simulink model "DCC_DTC_v3_5"  (R2023b)
settings: Solver=FixedStepDiscrete  StartTime=0.0  StopTime=0.4  MaxStep=1e-  RelTol=1e-6
undefined symbols (not defined in the file): DiscIntNeverNeededParam
libraries: spsPermanentMagnetSynchronousMachineLib x2, simulink x2, spsDCVoltageSourceLib x1, spsGroundLib x1, spsThreePhaseVIMeasurementLib x1, spsUniversalBridgeLib x1, sps_lib x1
settings Model: Creator=rainy  LastModifiedBy=rainy
settings DataIOCC: ReturnWorkspaceOutputs=off

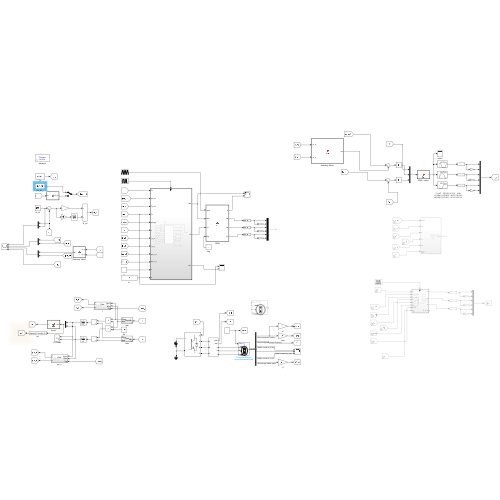
[thumbnail: Simulink's stored preview of the top-level diagram]
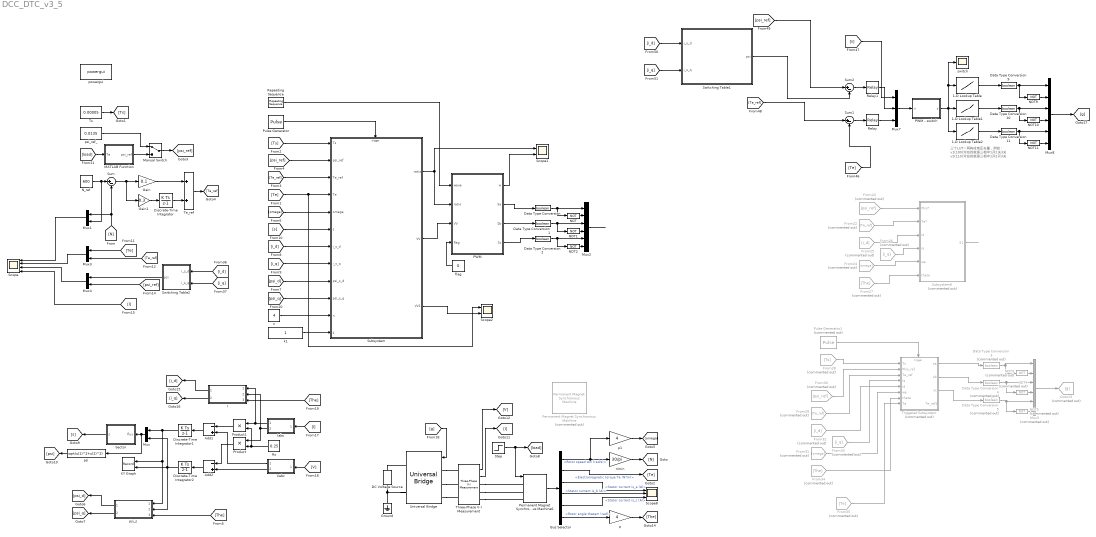
== system DCC_DTC_v3_5 ==
  note: 三个LUT一同构成电压矢量，例如：
      | v1(100)对应的就是三相中1开2关3关
      | v2(110)对应的就是三相中1开2开3关
  1-D Lookup Table : Lookup_n-D  NumberOfTableDimensions=1  BreakpointsForDimension1=[1 2 3 4 5 6]  Table=[1 1 0 0 0 1]  InternalRulePriority=Speed  RndMeth=Simplest
  1-D Lookup Table1 : Lookup_n-D  NumberOfTableDimensions=1  BreakpointsForDimension1=[1 2 3 4 5 6]  Table=[0 1 1 1 0 0]  InternalRulePriority=Speed  RndMeth=Simplest
  1-D Lookup Table2 : Lookup_n-D  NumberOfTableDimensions=1  BreakpointsForDimension1=[1 2 3 4 5 6]  Table=[0 0 0 1 1 1]  InternalRulePriority=Speed  RndMeth=Simplest
  Add1 : Sum  Inputs=-+
  Add2 : Sum  Inputs=-+
  Bus Selector : BusSelector  OutputSignals=Rotor speed wm (rad/s),Electromagnetic torque Te (N*m),Stator current is_a (A),Stator current is_b (A),Stator current is_c (A),Rotor angle thetam (rad)
  DC Voltage Source : spsDCVoltageSourceLib/DC Voltage Source  Amplitude=24  Measurements=Voltage
  Data Type Conversion{,1..2,9..11} (6 alike) : DataTypeConversion  OutDataTypeStr=boolean  SaturateOnIntegerOverflow=off  RndMeth=Floor
  Data Type Conversion3 : DataTypeConversion  Commented=on  OutDataTypeStr=boolean  SaturateOnIntegerOverflow=off  RndMeth=Floor
  Data Type Conversion4 : DataTypeConversion  Commented=on  OutDataTypeStr=boolean  SaturateOnIntegerOverflow=off  RndMeth=Floor
  Data Type Conversion5 : DataTypeConversion  Commented=on  OutDataTypeStr=boolean  SaturateOnIntegerOverflow=off  RndMeth=Floor
  Discrete-Time Integrator : DiscreteIntegrator  SampleTime=-1  ICPrevOutput=DiscIntNeverNeededParam  ICPrevScaledInput=DiscIntNeverNeededParam
  Discrete-Time Integrator1 : DiscreteIntegrator  SampleTime=-1  ICPrevOutput=DiscIntNeverNeededParam  ICPrevScaledInput=DiscIntNeverNeededParam
  Discrete-Time Integrator2 : DiscreteIntegrator  SampleTime=-1  ICPrevOutput=DiscIntNeverNeededParam  ICPrevScaledInput=DiscIntNeverNeededParam
  From22 : From  Commented=on  GotoTag=Te_ref
  From23 : From  Commented=on  GotoTag=psi_ref
  From24 : From  Commented=on  GotoTag=omega
  From25 : From  Commented=on  GotoTag=i_d
  From26 : From  Commented=on  GotoTag=i_q
  From27 : From  Commented=on  GotoTag=The
  From28 : From  Commented=on  GotoTag=Ts
  From29 : From  Commented=on  GotoTag=Te_ref
  From30 : From  Commented=on  GotoTag=psi_ref
  From31 : From  Commented=on  GotoTag=omega
  From32 : From  Commented=on  GotoTag=i_d
  From33 : From  Commented=on  GotoTag=i_q
  From34 : From  Commented=on  GotoTag=The
  From35 : From  Commented=on  GotoTag=Te
  Gain : Gain  Gain=0.1
  Gain1 : Gain  Gain=0.3
  Goto13 : Goto  Commented=on  GotoTag=g
  Ground : spsGroundLib/Ground  LConnTagsString=a
  I : Subsystem  ReferencedSubsystem=Park
  Iabc : Subsystem  ReferencedSubsystem=Clark
  MATLAB Function : MATLAB Function  TreatAsAtomicUnit=on
  Manual Switch : ManualSwitch
  Mux{,1,3..4} (4 alike) : Mux  Inputs=2
  Mux2 : Mux  Inputs=6
  Mux5 : Mux  Commented=on  Inputs=6
  Mux7 : Mux  Inputs=3
  Mux8 : Mux  Inputs=6
  NOT{,1..2,9..11} (6 alike) : Logic  Operator=NOT  IconShape=distinctive  AllPortsSameDT=off  OutDataTypeStr=boolean
  NOT3 : Logic  Commented=on  Operator=NOT  IconShape=distinctive  AllPortsSameDT=off  OutDataTypeStr=boolean
  NOT4 : Logic  Commented=on  Operator=NOT  IconShape=distinctive  AllPortsSameDT=off  OutDataTypeStr=boolean
  NOT5 : Logic  Commented=on  Operator=NOT  IconShape=distinctive  AllPortsSameDT=off  OutDataTypeStr=boolean
  N_ref : Constant  Value=600
  PWM : MATLAB Function  TreatAsAtomicUnit=on
  PWM - switch : MATLAB Function  TreatAsAtomicUnit=on
  Permanent Magnet Synchronous Machine : spsPermanentMagnetSynchronousMachineLib/Permanent Magnet Synchronous Machine  Commented=on  NbPhases=3  FluxDistribution=Sinusoidal  RotorType=Salient-pole  MechanicalLoad=Torque Tm  PresetModel="02:  1.7 Nm 300 Vdc 3750 RPM - 1.7 Nm"  ShowDetailedParameters=on  MeasurementBus=off  Resistance=4.765  Inductance=8.5e-3  dqInductances=[0.0133 0.0147]  La=0.0005  MachineConstant=Flux linkage established by magnets (V.s)  Flux=0.1848  VoltageCst=67.038  TorqueCst=0.5544  Flat=120  Mechanical=[0.0001051 4.047e-05 2 0]  PolePairs=2  InitialConditions=[0 0 0 0]  InitialConditions5ph=[0 0 0 0 0 0]  RefAngle=Aligned with phase A axis (original Park)  IterativeDiscreteModel=Trapezoidal non iterative  TsBlock=-1  TsPowergui=0
  Permanent Magnet Synchronous Machine6 : spsPermanentMagnetSynchronousMachineLib/Permanent Magnet Synchronous Machine  NbPhases=3  FluxDistribution=Sinusoidal  RotorType=Round  MechanicalLoad=Torque Tm  PresetModel=No  ShowDetailedParameters=on  MeasurementBus=off  Resistance=0.25  Inductance=8.5e-3  dqInductances=[8.5e-3,8.5e-3]  La=0.0005  MachineConstant=Flux linkage established by magnets (V.s)  Flux=0.01325  VoltageCst=9.6131  TorqueCst=0.0795  Flat=120  Mechanical=[0.00003 0 4 0]  PolePairs=4  InitialConditions=[0,0, 0,0]  InitialConditions5ph=[0 0 0 0 0 0]  RefAngle=Aligned with phase A axis (original Park)  IterativeDiscreteModel=Trapezoidal non iterative  TsBlock=-1  TsPowergui=0
  Product : Product
  Product1 : Product
  Pulse Generator : DiscretePulseGenerator  PulseType=Time based  Period=0.00005
  Pulse Generator1 : DiscretePulseGenerator  Commented=on  PulseType=Time based  Period=0.00005
  Relay : Relay  OnSwitchValue=0.01  OffSwitchValue=-0.01
  Relay1 : Relay  OnSwitchValue=0.0002  OffSwitchValue=-0.0002
  Repeating Sequence : simulink/Sources/Repeating Sequence  rep_seq_t=[0 0.000025 0.00005]  rep_seq_y=[0 1 0]
  Rs : Constant  Value=0.25
  Scope : Scope  NumInputPorts=4
  Scope1 : Scope  NumInputPorts=2
  Scope2 : Scope  NumInputPorts=2
  Scope8 : Scope  NumInputPorts=3
  Sector : MATLAB Function  TreatAsAtomicUnit=on
  Step : Step  Time=0.2  After=0.5  SampleTime=0
  Subsystem : Subsystem
  Subsystem6 : Subsystem  Commented=on
  Sum : Sum  Inputs=|+-
  Sum1 : Sum  Inputs=|+-
  Sum2 : Sum  Inputs=|+-
  Switching Table1 : MATLAB Function  TreatAsAtomicUnit=on
  Switching Table2 : MATLAB Function  TreatAsAtomicUnit=on
  Te_ref : Sum
  Three-Phase V-I Measurement : spsThreePhaseVIMeasurementLib/Three-Phase V-I Measurement  VoltageMeasurement=phase-to-ground  SetLabelV=off  LabelV=Vabc  Vpu=off  VpuLL=off  CurrentMeasurement=yes  SetLabelI=off  LabelI=Iabc  Ipu=off  Pbase=100e6  Vbase=500e3  OutputType=Complex  PhasorSimulation=off  PSBequivalent=0
  Triggered Subsystem : Subsystem  Commented=on  TreatAsAtomicUnit=on
  Ts : Constant  Value=0.00005
  Universal Bridge : spsUniversalBridgeLib/Universal Bridge  Arms=3  SnubberResistance=1e5  SnubberCapacitance=inf  Device=IGBT / Diodes  Ron=1e-3  Lon=0  ForwardVoltages="[  0  0  ]"  ForwardVoltage=0  GTOparameters=[ 10e-6 , 20e-6 ]  IGBTparameters=[ 1e-6 , 2e-6 ]  Measurements=None  Measurements_2=None  converterType=Rectifier
  Vabc : Subsystem  ReferencedSubsystem=Clark
  XY Graph : Record  FileSettingsInternal="{\"entries\":[{\"content\":{\"excelSettings\":{\"content\":{},\"type\":\"Streamout.ExcelSettings\"}},\"type\":\"Streamout.FileSettingStorage\",\"uuid\":\"\"}],\"packageUris\":[\"http:\\/\\/schema.mathworks.com\\/mf0\\/streamout_blocks\\/R2020a\"],\"version\":\"1.0\"}"  Layout=[1 1]  SignalsInternal="{\"entries\":[{\"content\":{\"signals\":[{\"content\":{\"blockPath\":[],\"dimensions\":[1],\"domain\":\"\",\"lineColor\":\"#a2142f\",\"plots\":[1],\"port\":1,\"sid\":[\"\"],\"signalID\":13639,\"signalName\":\"Discrete-Time\\nIntegrator1\"},\"type\":\"RecordBlkView.Signal\",\"uuid\":\"\"},{\"content\":{\"blockPath\":[],\"dimensions\":[1],\"domain\":\"\",\"lineColor\":\"#139fff\",\"plots\":[1],\"port\":2,\"sid\":[\"\"],\"signalID\":13643,\"signalName\":\"Discrete-Time\\nIntegrator2\"},\"type\":\"RecordBlkView.Signal\",\"uuid\":\"\"}]},\"type\":\"RecordBlkView.InputSignals\",\"uuid\":\"\"}],\"packageUris\":[\"http:\\/\\/schema.mathworks.com\\/mf0\\/streamout_blocks\\/R2020a\"],\"version\":\"1.0\"}"  VisualizationBindings="{\"xyplotplugin\":{\"info\":[{\"series\":[{\"bindingParametersList\":[{\"parameter\":\"X-Axis\",\"signalID\":13639,\"signalName\":\"Discrete-Time\\nIntegrator1\"},{\"parameter\":\"Y-Axis\",\"signalID\":13643,\"signalName\":\"Discrete-Time\\nIntegrator2\"}],\"seriesID\":35459}],\"subplotID\":1}]}}"  CompatibilityTag=XY  st=-1
  flag : Constant  Value=0
  k1 : Constant
  n : Constant  Value=4
  p : Gain  Gain=4
  p1 : Gain  Gain=4
  powergui : sps_lib/powergui  Priority=1  SimulationMode=Discrete  SampleTime=1e-6  frequency=60  Iterations=50  frequencyindice=0  Pbase=100e6  ErrMax=1e-4  UnitsV=kV  UnitsW=MW  buscounter=0  FunctionMessages=off  echomessages=off  EnableUseOfTLC=off  CurrentSourceSwitches=off  DisableSnubberDevices=off  DisableRonSwitches=off  DisableVfSwitches=off  DisplayEquations=off  AutomaticDiscreteSolvers=off  SolverType=Tustin/Backward Euler (TBE)  Interpol=off  ExternalGateDelay=off  methode=off  Ts=100  x0status=blocks  SPID=on  SwTol=0  HookPort=off  NonlinearTolerance=1e-4  nMaxIteration=100  ContinueOnMaxIteration=off  RestoreLinks=warning  ResistiveCurrentMeasurement=off  Frange=[0:2:500]  Ylog=off  Xlog=on  ShowGrid=off  save=off  variable=ZData  structure=0  ZoomFFT=off  StartTime=0.0  cycles=1  DisplayStyle=1  fundamental=60  FreqAxis=off  MaxFrequency=1000  frequencyindicesteady=1  RmsSteady=1  display=off
  psi : Fcn  Expr=sqrt(u(1)^2+u(2)^2)
  psi_ref_ : Constant  Value=0.0135
  psi_s : Subsystem  ReferencedSubsystem=Park
  r/min : Gain  Gain=30/pi
  switch : Scope
  wires:
  N_ref/1 -> Mux1/2, Sum/1
  Sum/1 -> Gain/1, Gain1/1
  Gain1/1 -> Discrete-Time Integrator/1
  Gain/1 -> Te_ref/1
  Bus Selector/1 -> p1/1, r/min/1  "<Rotor speed wm (rad/s)>"
  r/min/1 -> [N]
  [N] -> Sum/2, Mux1/1
  NOT1/1 -> Mux2/4
  Data Type Conversion2/1 -> NOT2/1, Mux2/5
  NOT2/1 -> Mux2/6
  Data Type Conversion/1 -> NOT/1, Mux2/1
  NOT/1 -> Mux2/2
  Data Type Conversion1/1 -> NOT1/1, Mux2/3
  Iabc/1 -> I/1, Product1/1
  Iabc/2 -> Product/1, I/2
  Rs/1 -> Product/2, Product1/2
  Product1/1 -> Add1/1
  Vabc/1 -> Add1/2
  Product/1 -> Add2/1
  Vabc/2 -> Add2/2
  Add2/1 -> Discrete-Time Integrator2/1
  Add1/1 -> Discrete-Time Integrator1/1
  Ts/1 -> [Ts]
  Mux/1 -> psi/1, Sector/1(flux)
  Bus Selector/2 -> [Te]  "<Electromagnetic torque Te (N*m)>"
  [Te] -> Scope2/1, Subsystem/4(Te)
  Three-Phase V-I Measurement/2 -> [I]
  Discrete-Time Integrator/1 -> Te_ref/2
  PWM/4(Sc) -> Data Type Conversion2/1
  PWM/3(Sb) -> Data Type Conversion1/1
  PWM/2(Sa) -> Data Type Conversion/1
  [Ts] -> Subsystem/1(Ts)
  [psi_ref] -> Subsystem/2(psi_ref)
  Repeating Sequence/1 -> PWM/1(wave)
  Pulse Generator/1 -> Subsystem/Trigger
  n/1 -> Subsystem/11(n)
  flag/1 -> PWM/4(flag)
  Bus Selector/3 -> Scope8/1  "<Stator current is_a (A)>"
  Bus Selector/4 -> Scope8/2  "<Stator current is_b (A)>"
  Bus Selector/5 -> Scope8/3  "<Stator current is_c (A)>"
  Step/1 -> Permanent Magnet Synchronous Machine6/1, [load]
  Subsystem/1(ratio) -> PWM/2(ratio), Scope1/1
  Subsystem/2(VV) -> PWM/3(VV)
  Te_ref/1 -> [Te_ref]
  [Te_ref] -> Subsystem/3(Te_ref)
  [omega] -> Subsystem/5(omega)
  [i_d] -> Subsystem/7(i_s_d)
  [i_q] -> Subsystem/8(i_s_q)
  Sector/1(s) -> [s]
  [s] -> Subsystem/6(s)
  PWM/1(w) -> Scope1/2
  psi/1 -> [psi]
  Mux1/1 -> Scope/1
  Mux3/1 -> Scope/2
  Mux4/1 -> Scope/3
  [I] -> Scope/4
  [Te] -> Mux3/1
  Switching Table2/1(psi) -> Mux4/1
  [Te_ref] -> Mux3/2
  [psi_ref] -> Mux4/2
  Three-Phase V-I Measurement/1 -> [V]
  [I] -> Iabc/1
  [V] -> Vabc/1
  Mux2/1 -> ?
  [g] -> Universal Bridge/1
  Bus Selector/6 -> p/1  "<Rotor angle thetam (rad)>"
  p/1 -> [The]
  [The] -> I/3
  I/2 -> [i_q]
  I/1 -> [i_d]
  p1/1 -> [omega]
  k1/1 -> Subsystem/12(k)
  psi_s/1 -> [psi_d]
  Discrete-Time Integrator1/1 -> XY Graph/1, psi_s/1, Mux/1
  psi_s/2 -> [psi_q]
  [The] -> psi_s/3
  Discrete-Time Integrator2/1 -> psi_s/2, XY Graph/2, Mux/2
  [psi_q] -> Subsystem/10(psi_s_q)
  [psi_d] -> Subsystem/9(psi_s_d)
  [load] -> MATLAB Function/1(Te)
  psi_ref_/1 -> Manual Switch/1
  MATLAB Function/1(psi_ref) -> Manual Switch/2
  Manual Switch/1 -> [psi_ref]
  From23/1 -> Subsystem6/1(Phis*)
  From22/1 -> Subsystem6/2(Te*)
  From25/1 -> Subsystem6/3(id)
  From24/1 -> Subsystem6/5(we)
  From26/1 -> Subsystem6/4(iq)
  From27/1 -> Subsystem6/6("theta ")
  NOT5/1 -> Mux5/6
  Triggered Subsystem/2(sb) -> Data Type Conversion4/1
  Data Type Conversion5/1 -> NOT5/1, Mux5/5
  Data Type Conversion4/1 -> NOT4/1, Mux5/3
  Triggered Subsystem/3(sc) -> Data Type Conversion5/1
  Triggered Subsystem/1(sa) -> Data Type Conversion3/1
  NOT4/1 -> Mux5/4
  Data Type Conversion3/1 -> NOT3/1, Mux5/1
  NOT3/1 -> Mux5/2
  Pulse Generator1/1 -> Triggered Subsystem/Trigger
  From28/1 -> Triggered Subsystem/1(Ts)
  From31/1 -> Triggered Subsystem/6(we)
  From29/1 -> Triggered Subsystem/3(Te_ref)
  From34/1 -> Triggered Subsystem/7(theta)
  From32/1 -> Triggered Subsystem/5(id)
  From30/1 -> Triggered Subsystem/2(Phis_ref)
  From33/1 -> Triggered Subsystem/4(iq)
  Permanent Magnet Synchronous Machine6/1 -> Bus Selector/1
  Subsystem6/1(S1) -> ?
  Mux5/1 -> Goto13/1
  Subsystem/3(VV1) -> Scope2/2
  From35/1 -> Triggered Subsystem/8(Te)
  PWM - switch/1(y) -> 1-D Lookup Table2/1, switch/1, 1-D Lookup Table/1, 1-D Lookup Table1/1
  Relay1/1 -> Mux7/2
  Relay/1 -> Mux7/3
  Data Type Conversion9/1 -> NOT9/1, Mux8/1
  1-D Lookup Table2/1 -> Data Type Conversion11/1
  Mux7/1 -> PWM - switch/1(u)
  Sum2/1 -> Relay1/1
  1-D Lookup Table/1 -> Data Type Conversion9/1
  NOT10/1 -> Mux8/4
  NOT9/1 -> Mux8/2
  Data Type Conversion10/1 -> Mux8/3, NOT10/1
  1-D Lookup Table1/1 -> Data Type Conversion10/1
  Sum1/1 -> Relay/1
  Data Type Conversion11/1 -> Mux8/5, NOT11/1
  NOT11/1 -> Mux8/6
  Mux8/1 -> [g]
  [s] -> Mux7/1
  [psi_ref] -> Sum2/1
  [Te] -> Sum1/2
  [Te_ref] -> Sum1/1
  Switching Table1/1(psi) -> Sum2/2
  [i_d] -> Switching Table1/1(i_s_d)
  [i_q] -> Switching Table1/2(i_s_q)
  [i_d] -> Switching Table2/1(i_s_d)
  [i_q] -> Switching Table2/2(i_s_q)
  connections:
  Universal Bridge/RConn2 -- DC Voltage Source/LConn1 -- Ground/LConn1
  Universal Bridge/LConn3 -- Three-Phase V-I Measurement/LConn3
  Universal Bridge/LConn1 -- Three-Phase V-I Measurement/LConn1
  Universal Bridge/LConn2 -- Three-Phase V-I Measurement/LConn2
  DC Voltage Source/RConn1 -- Universal Bridge/RConn1
  Three-Phase V-I Measurement/RConn1 -- Permanent Magnet Synchronous Machine6/LConn1
  Three-Phase V-I Measurement/RConn2 -- Permanent Magnet Synchronous Machine6/LConn2
  Three-Phase V-I Measurement/RConn3 -- Permanent Magnet Synchronous Machine6/LConn3

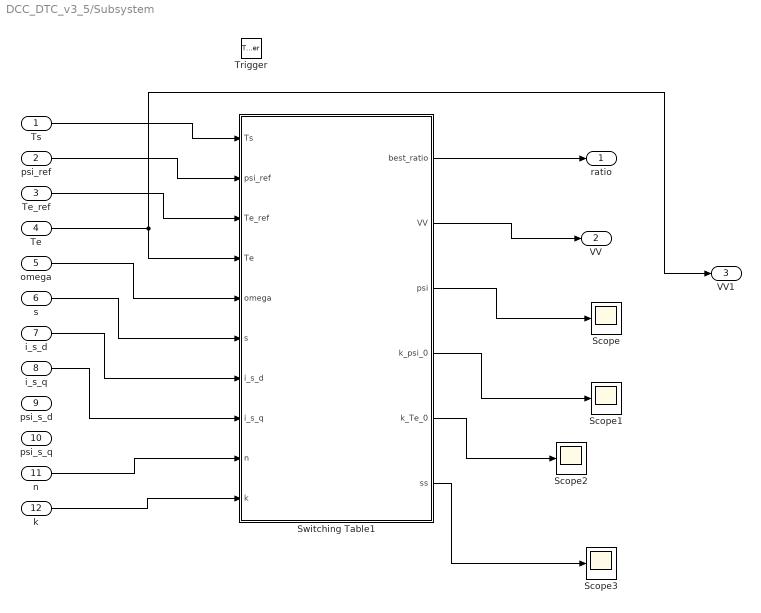
== system DCC_DTC_v3_5/Subsystem ==
  Ts : Inport
  psi_ref : Inport  Port=2
  Te_ref : Inport  Port=3
  Te : Inport  Port=4
  omega : Inport  Port=5
  s : Inport  Port=6
  i_s_d : Inport  Port=7
  i_s_q : Inport  Port=8
  psi_s_d : Inport  Port=9
  psi_s_q : Inport  Port=10
  n : Inport  Port=11
  k : Inport  Port=12
  Trigger : TriggerPort  VariantControl=(inherit)  PortDimensions=1
  Scope{,1..3} (4 alike) : Scope
  Switching Table1 : MATLAB Function  TreatAsAtomicUnit=on
  ratio : Outport
  VV : Outport  Port=2
  VV1 : Outport  Port=3
  wires:
  Ts/1 -> Switching Table1/1(Ts)
  psi_ref/1 -> Switching Table1/2(psi_ref)
  Te_ref/1 -> Switching Table1/3(Te_ref)
  Te/1 -> Switching Table1/4(Te), VV1/1
  omega/1 -> Switching Table1/5(omega)
  s/1 -> Switching Table1/6(s)
  i_s_q/1 -> Switching Table1/8(i_s_q)
  Switching Table1/1(best_ratio) -> ratio/1
  k/1 -> Switching Table1/10(k)
  n/1 -> Switching Table1/9(n)
  Switching Table1/2(VV) -> VV/1
  i_s_d/1 -> Switching Table1/7(i_s_d)
  Switching Table1/3(psi) -> Scope/1
  Switching Table1/4(k_psi_0) -> Scope1/1
  Switching Table1/5(k_Te_0) -> Scope2/1
  Switching Table1/6(ss) -> Scope3/1

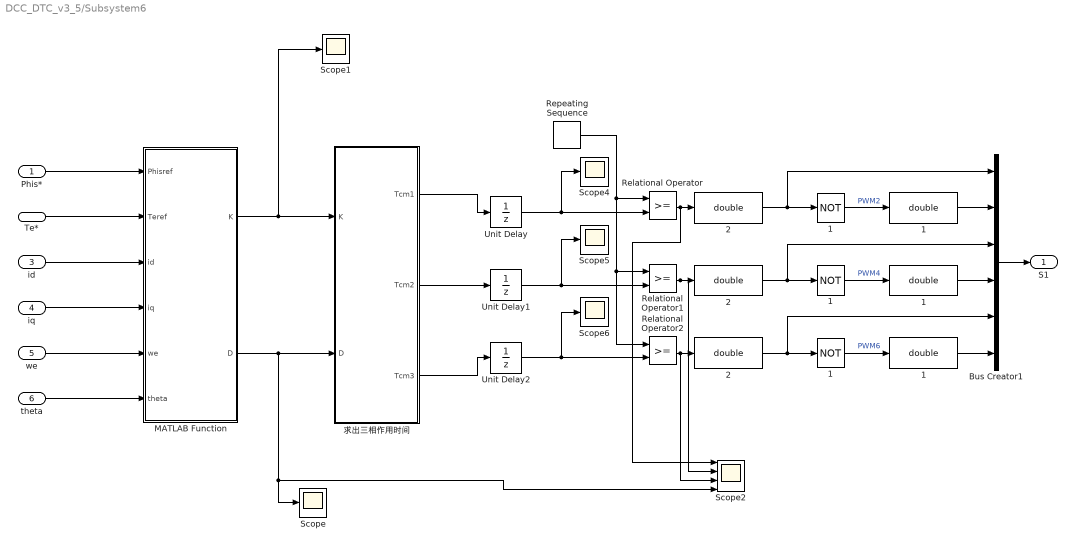
== system DCC_DTC_v3_5/Subsystem6 ==
  Phis* : Inport
  Te* : Inport  Port=2
  id : Inport  Port=3
  iq : Inport  Port=4
  we : Inport  Port=5
  "theta " : Inport  Port=6
  "         1" : DataTypeConversion  OutDataTypeStr=double  SaturateOnIntegerOverflow=off  RndMeth=Floor
  "         2" : DataTypeConversion  OutDataTypeStr=double  SaturateOnIntegerOverflow=off  RndMeth=Floor
  "       1" : Logic  Operator=NOT  AllPortsSameDT=off  OutDataTypeStr=boolean
  "     1" : DataTypeConversion  OutDataTypeStr=double  SaturateOnIntegerOverflow=off  RndMeth=Floor
  "     2" : DataTypeConversion  OutDataTypeStr=double  SaturateOnIntegerOverflow=off  RndMeth=Floor
  "   1" : Logic  Operator=NOT  AllPortsSameDT=off  OutDataTypeStr=boolean
  "  1" : DataTypeConversion  OutDataTypeStr=double  SaturateOnIntegerOverflow=off  RndMeth=Floor
  "  2" : DataTypeConversion  OutDataTypeStr=double  SaturateOnIntegerOverflow=off  RndMeth=Floor
  " 1" : Logic  Operator=NOT  AllPortsSameDT=off  OutDataTypeStr=boolean
  Bus Creator1 : BusCreator  Inputs=6
  MATLAB Function : MATLAB Function  TreatAsAtomicUnit=on
  Relational Operator : RelationalOperator  OutDataTypeStr=boolean  RndMeth=Simplest  InputSameDT=off
  Relational Operator1 : RelationalOperator  OutDataTypeStr=boolean  RndMeth=Simplest  InputSameDT=off
  Relational Operator2 : RelationalOperator  OutDataTypeStr=boolean  RndMeth=Simplest  InputSameDT=off
  Repeating Sequence : simulink/Sources/Repeating Sequence  rep_seq_t=[0 0.000025 0.00005]  rep_seq_y=[0 0.000025 0]
  Scope{,1,4..6} (5 alike) : Scope
  Scope2 : Scope  NumInputPorts=4
  Unit Delay : UnitDelay  SampleTime=0.00005  HasFrameUpgradeWarning=on
  Unit Delay1 : UnitDelay  SampleTime=0.00005  HasFrameUpgradeWarning=on
  Unit Delay2 : UnitDelay  SampleTime=0.00005  HasFrameUpgradeWarning=on
  求出三相作用时间 : MATLAB Function  TreatAsAtomicUnit=on
  S1 : Outport  VectorParamsAs1DForOutWhenUnconnected=off
  wires:
  Phis*/1 -> MATLAB Function/1(Phisref)
  Te*/1 -> MATLAB Function/2(Teref)
  id/1 -> MATLAB Function/3(id)
  iq/1 -> MATLAB Function/4(iq)
  we/1 -> MATLAB Function/5(we)
  "theta "/1 -> MATLAB Function/6(theta)
  MATLAB Function/1(K) -> Scope1/1, 求出三相作用时间/1(K)
  MATLAB Function/2(D) -> Scope2/4, Scope/1, 求出三相作用时间/2(D)
  求出三相作用时间/3(Tcm3) -> Unit Delay2/1
  "   1"/1 -> "     1"/1  "PWM4"
  "     2"/1 -> Bus Creator1/3, "   1"/1
  "     1"/1 -> Bus Creator1/4
  求出三相作用时间/1(Tcm1) -> Unit Delay/1
  " 1"/1 -> "  1"/1  "PWM2"
  Repeating Sequence/1 -> Relational Operator2/1, Relational Operator1/1, Relational Operator/1
  Relational Operator/1 -> Scope2/1, "  2"/1
  Relational Operator1/1 -> Scope2/2, "     2"/1
  求出三相作用时间/2(Tcm2) -> Unit Delay1/1
  "  1"/1 -> Bus Creator1/2
  "         2"/1 -> Bus Creator1/5, "       1"/1
  Relational Operator2/1 -> Scope2/3, "         2"/1
  "       1"/1 -> "         1"/1  "PWM6"
  "  2"/1 -> Bus Creator1/1, " 1"/1
  Bus Creator1/1 -> S1/1
  "         1"/1 -> Bus Creator1/6
  Unit Delay/1 -> Relational Operator/2, Scope4/1
  Unit Delay1/1 -> Scope5/1, Relational Operator1/2
  Unit Delay2/1 -> Relational Operator2/2, Scope6/1

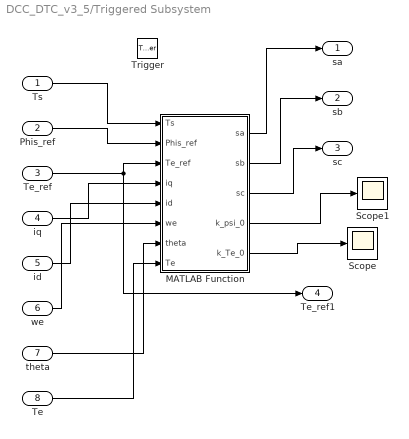
== system DCC_DTC_v3_5/Triggered Subsystem ==
  Ts : Inport
  Phis_ref : Inport  Port=2
  Te_ref : Inport  Port=3
  iq : Inport  Port=4
  id : Inport  Port=5
  we : Inport  Port=6
  theta : Inport  Port=7
  Te : Inport  Port=8
  Trigger : TriggerPort  VariantControl=(inherit)
  MATLAB Function : MATLAB Function  TreatAsAtomicUnit=on
  Scope : Scope
  Scope1 : Scope
  sa : Outport
  sb : Outport  Port=2
  sc : Outport  Port=3
  Te_ref1 : Outport  Port=4
  wires:
  Phis_ref/1 -> MATLAB Function/2(Phis_ref)
  Te_ref/1 -> Te_ref1/1, MATLAB Function/3(Te_ref)
  iq/1 -> MATLAB Function/4(iq)
  id/1 -> MATLAB Function/5(id)
  we/1 -> MATLAB Function/6(we)
  theta/1 -> MATLAB Function/7(theta)
  MATLAB Function/1(sa) -> sa/1
  MATLAB Function/2(sb) -> sb/1
  MATLAB Function/3(sc) -> sc/1
  Ts/1 -> MATLAB Function/1(Ts)
  Te/1 -> MATLAB Function/8(Te)
  MATLAB Function/5(k_Te_0) -> Scope/1
  MATLAB Function/4(k_psi_0) -> Scope1/1

== matlab function DCC_DTC_v3_5/PWM - switch ==
  data: u input; y output
function y = fcn(u)

% u(1) 扇区
% u(2) 磁链
% u(3) 转矩

V_Table=[5 6 1 2 3 4;3 4 5 6 1 2;6 1 2 3 4 5;2 3 4 5 6 1];
x=2*u(2)+u(3)+1;

y = V_Table(x, u(1));

== matlab function DCC_DTC_v3_5/Switching Table2 ==
  data: i_s_d input; i_s_q input; psi output
function psi = fcn(i_s_d, i_s_q)

% 给定的参数值
p = 4;
R_s = 0.25;
L_d = 0.0005;
L_q = 0.0005;
V = 24;
psi_f = 0.01325;

psi_r = psi_f + 1i*0;
psi_s_d = L_d*i_s_d + psi_f;
psi_s_q = L_q*i_s_q;

i_s = i_s_d + 1i*i_s_q;
psi_s = psi_s_d + 1i*psi_s_q;


% 计算零电压矢量下变化率
psi = sqrt(psi_s_d^2 +psi_s_q^2)

== matlab function DCC_DTC_v3_5/Switching Table1 ==
  data: i_s_d input; i_s_q input; psi output
function psi = fcn(i_s_d, i_s_q)

% 给定的参数值
p = 4;
R_s = 0.25;
L_d = 0.0005;
L_q = 0.0005;
V = 24;
psi_f = 0.01325;

psi_r = psi_f + 1i*0;
psi_s_d = L_d*i_s_d + psi_f;
psi_s_q = L_q*i_s_q;

i_s = i_s_d + 1i*i_s_q;
psi_s = psi_s_d + 1i*psi_s_q;


% 计算零电压矢量下变化率
psi = sqrt(psi_s_d^2 +psi_s_q^2)

== matlab function DCC_DTC_v3_5/Sector ==
  data: flux input; s output
function s = fcn(flux)

% 将\psi_{\aplha}和\psi_{\beta}分解为三相
a1 = flux(1);
b1 = flux(1)*(-0.5) + sqrt(3)/2*flux(2);
c1 = flux(1)*(-0.5) - sqrt(3)/2*flux(2);

% a1 > 0，有扇区126
% b1 > 0，有扇区234
% c1 > 0，有扇区456
% n为a1 b1 c1中>0的个数，0 < n < 3
% 
% a b c | s
%-------|---
% 1 1 0 | 2
% 1 0 1 | 6
% 1 0 0 | 1
% 0 1 1 | 4
% 0 1 0 | 3
% 0 0 1 | 5

if(flux(2) == 0)
    N = 4;
else
    if(a1 > 0)
        a = 1;
    else
        a = 0;
    end
    
    if(b1 > 0)
        b = 1;
    else
        b = 0;
    end
    
    if(c1 > 0)
        c = 1;
    else
        c = 0;
    end
    
    N = 4*a+2*b+c;
end

% if(N==0 || N==7)
%     N = 4;
% end

Sector_table=[5 3 4 1 6 2];

s = Sector_table(N);

== matlab function DCC_DTC_v3_5/PWM ==
  data: w output; wave input; ratio input; VV input; Sa output; Sb output; Sc output; flag input
function [w, Sa, Sb, Sc] = fcn(wave, ratio, VV, flag)

sw = [1 0 0; 1 1 0; 0 1 0; 0 1 1; 0 0 1; 1 0 1];

if(VV<1 || VV>6)
    VV = 1;
end

if(wave >= 1 - ratio || flag == 0)
    Sa= sw(VV, 1);
    Sb= sw(VV, 2);
    Sc= sw(VV, 3);
    w = 1;
else
    Sa = 0;
    Sb = 0;
    Sc = 0;
    w = 0;
end

== matlab function DCC_DTC_v3_5/Subsystem6/求出三相作用时间 ==
  settings: updateMethod=DISCRETE  sampleTime=0.00005
  data: K input; Tcm1 output; D input; Tcm2 output; Tcm3 output
function [Tcm1,Tcm2,Tcm3] = fcn(K,D)

Ts=0.00005;

T1=D*Ts/2;
T2=T1;
Ta=(Ts-T1-T2)/4;
Tb=Ta+T1/2;
Tc=Tb+T2/2;
Tcm1=1;
Tcm2=1;
Tcm3=1;

if(K==1)
    Tcm1=Tc;Tcm2=Tc;Tcm3=Tc;
end
if(K==2) 
    Tcm1=Ta;Tcm2=Tc;Tcm3=Tc;
end
if(K==3) 
    Tcm1=Ta;Tcm2=Ta;Tcm3=Tc;
end
if(K==4) 
    Tcm1=Tc;Tcm2=Ta;Tcm3=Tc;
end
if(K==5) 
    Tcm1=Tc;Tcm2=Ta;Tcm3=Ta;
end
if(K==6) 
    Tcm1=Tc;Tcm2=Tc;Tcm3=Ta;
end
if(K==7) 
    Tcm1=Ta;Tcm2=Tc;Tcm3=Ta;
end
if(K==8)
    Tcm1=Ta;Tcm2=Ta;Tcm3=Ta;
end

== matlab function DCC_DTC_v3_5/Subsystem/Switching Table1 ==
  data: best_ratio output; Ts input; psi_ref input; Te_ref input; Te input; VV output; omega input; s input; i_s_d input; i_s_q input; n input; k input; psi output; k_psi_0 output; k_Te_0 output; ss output
function [best_ratio, VV, psi, k_psi_0, k_Te_0, ss]= fcn(Ts, psi_ref, Te_ref, Te, omega, s, i_s_d, i_s_q, n, k)

% 给定的参数值
p = 4;
R_s = 0.25;
L_d = 0.0005;
L_q = 0.0005;
V = 24;
psi_f = 0.01325;

psi_r = psi_f + 1i*0;
psi_s_d = L_d*i_s_d + psi_f;
psi_s_q = L_q*i_s_q;

i_s = i_s_d + 1i*i_s_q;
psi_s = psi_s_d + 1i*psi_s_q;


% 计算零电压矢量下变化率
psi = sqrt(psi_s_d^2 +psi_s_q^2);
k_psi_0 = -R_s/psi*real(psi_s'*i_s); % 零电压矢量时磁链变化率
% k_psi_1 = 1/psi*real(psi_s'*u_s) + k_psi_0; % 非零电压矢量时磁链变化率

k_Te_0 = -3/2*p*(1/L_q-1/L_d)*omega*real(psi_s^2) + ...
    3/4*p*R_s*(1/L_d^2-1/L_q^2)*imag(psi_s^2) - ...
    3/2*p/L_d*(R_s/L_d*imag(psi_s*psi_r) + omega*real(psi_s*psi_r)); % 零电压矢量时转矩变化率
ss = psi_s*psi_r;
% k_Te_1 = 3/2*p*(1/L_q-1/L_d)*imag(u_s*psi_s) + 3/2*p/L_d*imag(u_s*psi_r) + k_Te_0;  % 非零电压矢量时转矩变化率



% 选择电压矢量
Te1 = Te + k_Te_0*Ts;
psi1 = psi + k_psi_0*Ts;

if(Te_ref > Te1)
    if(psi_ref > psi)
        VV = s+1;
    else
        VV = s+2;
    end
else
    if(psi_ref > psi)
        VV = s-1;
    else
        VV = s-2;
    end
end

if(VV < 1)
    VV = VV+6;
end
if(VV > 6)
    VV = VV-6;
end


% MPTC
u_s = cos(pi/6*(VV-1))*V + 1i*sin(pi/6*(VV-1))*V;
k_psi_1 = 1/psi*real(psi_s'*u_s) + k_psi_0; % 非零电压矢量时磁链变化率
k_Te_1 = 3/2*p*(1/L_q-1/L_d)*imag(u_s*psi_s) + 3/2*p/L_d*imag(u_s*psi_r) + k_Te_0;  % 非零电压矢量时转矩变化率

g_min = Inf;
best_ratio = 1;

d_Te = 0;
d_psi = 0;

for i=1:n+1
    ratio = (i-1)*1/n;

    Te1_ = Te + Ts*ratio*k_Te_1 + Ts*(1-ratio)*k_Te_0;
    psi_s1 = psi_s + Ts*ratio*k_psi_1 + Ts*(1-ratio)*k_psi_0;

    d_Te = abs(Te_ref - Te1_);
    d_psi = k*abs(psi_ref - abs(psi_s1));

    g = d_Te + d_psi;

    if(g < g_min)
        g_min = g;
        best_ratio =ratio;
    end
end

== matlab function DCC_DTC_v3_5/MATLAB Function ==
  data: Te input; psi_ref output
function psi_ref = fcn(Te)

p = 2;
R_s = 4.765;
L_d = 0.0133;
L_q = 0.0147;
V = 300;
psi_f = 0.1848;

psi_ref = sqrt(psi_f^2 + ((2*L_q)/(3*p*psi_f))^2);

== matlab function DCC_DTC_v3_5/Subsystem6/MATLAB Function ==
  settings: updateMethod=DISCRETE  sampleTime=0.00005
  data: Phisref input; Teref input; id input; iq input; we input; theta input; K output; D output
function [K,D]  = fcn(Phisref,Teref,id,iq,we,theta)

% Ts=0.00005;R=4.765;Ld=0.0133;Lq=0.0147;Phif=0.1848;p=2;Vdc=300;gmin=20000000000000;m=250;K=1;D=1;
Ts=0.00005;R=0.25;Ld=0.0005;Lq=0.0005;Phif=0.01325;p=4;Vdc=24;gmin=20000000000000;m=250;K=1;D=1;

sw=[0 0 0;1 0 0;1 1 0;0 1 0;0 1 1;0 0 1;1 0 1;1 1 1];
trans=2/3*[cos(theta) cos(theta-2*pi/3) cos(theta+2*pi/3);-sin(theta) -sin(theta-2*pi/3) -sin(theta+2*pi/3)];


persistent M ud22 uq22 
if isempty(M)
    M=1; 
    ud22=0;  
    uq22=0; 
end

iq1=iq;
id1=id;
Te=3/2*p*iq1*Phif;
for i=1:8
      sa=sw(i,1);sb=sw(i,2);sc=sw(i,3);
      Va=(Vdc*(2*sa-sb-sc))/3;
      Vb=(Vdc*(2*sb-sa-sc))/3;   
      Vc=(Vdc*(2*sc-sb-sa))/3;
      Vabc=[Va;Vb;Vc];
      Vdq=trans*Vabc;
      Vd=Vdq(1,1);
      Vq=Vdq(2,1);
      idid=1/Ld*(Vd-R*id1+we*Lq*iq1)*Ts;
      iqid=1/Lq*(Vq-R*iq1-we*(Phif+Ld*id1))*Ts;
      idnext=id1+idid;
      iqnext=iq1+iqid;
      Tenext=3/2*p*iqnext*Phif;
      Phidnext=Ld*idnext+Phif;
      Phiqnext=Lq*iqnext;
      Phisnext=(Phidnext*Phidnext+Phiqnext*Phiqnext)^(1/2);
      
      ST0=1/Lq*(-R*iq1-we*(Phif+Ld*id1))*(3/2*p*Phif);
      STi=1/Lq*(Vq-R*iq1-we*(Phif+Ld*id1))*(3/2*p*Phif);
      Di=(Teref-Te-ST0*Ts)/(STi-ST0)/Ts;
      
      if(Di<=0||Di>=1)
          D_flag=100000;
          Di=1;
      else
          D_flag=0;
      end
      
      g=abs(Teref-Tenext)+m*abs(Phisref-Phisnext)+D_flag;
     
       if(g<gmin)
        K=i;
        D=Di;
        gmin=g;
      end
end

sa=sw(K,1);sb=sw(K,2);sc=sw(K,3);
Vamin=(Vdc*(2*sa-sb-sc))/3;
Vbmin=(Vdc*(2*sb-sa-sc))/3;   
Vcmin=(Vdc*(2*sc-sb-sa))/3;
Vabcmin=[Vamin;Vbmin;Vcmin];
Vdqmin=trans*Vabcmin;
ud22=Vdqmin(1,1)*D;
uq22=Vdqmin(2,1)*D;

== matlab function DCC_DTC_v3_5/Triggered Subsystem/MATLAB Function ==
  data: Ts input; Phis_ref input; sa output; Te_ref input; iq input; id input; we input; theta input; sb output; sc output; Te input; k_psi_0 output; k_Te_0 output
function [sa, sb, sc, k_psi_0, k_Te_0] = fcn(Ts, Phis_ref, Te_ref, iq, id, we, theta, Te)

R       = 0.25;
Ld      = 0.0005;
Lq      = 0.0005;
Phif    = 0.01325;
p       = 4;
Vdc     = 24;
gmin    = 20000000;
m       = 50;
imin    = 1;

sw = [0 0 0; 0 0 1; 0 1 0; 0 1 1; 1 0 0; 1 0 1; 1 1 0; 1 1 1];
trans = 2/3*[cos(theta) cos(theta-2/3*pi) cos(theta+2/3*pi);
             -sin(theta) -sin(theta-2/3*pi) -sin(theta+2/3*pi)];

persistent flag ud_prev uq_prev ud_next uq_next
if isempty(flag)
    flag = 1;
    ud_prev = 0;
    uq_prev = 0;
    ud_next = 0;
    uq_next = 0;
end

ud_prev = ud_next;
uq_prev = uq_next;

R_s=R;
L_d=Ld;
L_q=Lq;
psi_f=Phif;
omega=we;

i_s_d = id;
i_s_q = iq;
psi_s_d = L_d*i_s_d + psi_f;
psi_s_q = L_q*i_s_q;

i_s = i_s_d + 1i*i_s_q;
psi_s = psi_s_d + 1i*psi_s_q;
psi_r = psi_f + 1i*0;

% 计算零电压矢量下变化率
psi = sqrt(psi_s_d^2 +psi_s_q^2);
k_psi_0 = -R_s/psi*real(psi_s'*i_s); % 零电压矢量时磁链变化率

k_Te_0 = -3/2*p*(1/L_q-1/L_d)*omega*real(psi_s^2) + ...
    3/4*p*R_s*(1/L_d^2-1/L_q^2)*imag(psi_s^2) - ...
    3/2*p/L_d*(R_s/L_d*imag(psi_s*psi_r) + omega*real(psi_s*psi_r)); % 零电压矢量时转矩变化率

% 选择电压矢量
Te1 = Te + k_Te_0*Ts;
psi1 = psi + k_psi_0*Ts;

% id1 = id+Ts/Ld*(ud_prev+iq*we*Lq-id*R);
% iq1 = iq+Ts/Lq*(uq_prev-id*we*Ld-iq*R-Phif*we);

id1 = id;
iq1 = iq;

for i=1:8
    sa = sw(i,1); sb = sw(i, 2); sc = sw(i, 3);
    Va = Vdc*(2*sa-sb-sc)/3;
    Vb = Vdc*(2*sb-sc-sa)/3;
    Vc = Vdc*(2*sc-sa-sb)/3;
    Vabc = [Va; Vb; Vc];
    Vdq = trans*Vabc;
    Vd = Vdq(1, 1);
    Vq = Vdq(2, 1);
    id2 = id1+Ts/Ld*(Vd+iq1*we*Lq-id1*R);
    iq2 = iq1+Ts/Lq*(Vq-id1*we*Ld-iq1*R-Phif*we);
    Te2 = 3/2*p*iq2*Phif;
    Phid2 = Ld*id2+Phif;
    Phiq2 = Lq*iq2;
    Phis2 = (Phid2^2+Phiq2^2)^0.5;
    d_Te = abs(Te_ref - Te2);
    d_Phis = abs(Phis_ref-Phis2);
    g = abs(Te_ref - Te2)+m*abs(Phis_ref-Phis2);
    [i g d_Te m*d_Phis];
    if i==1
        [Te1 Te2 psi1 Phis2];
    end
    if (g<gmin)
        imin = i;
        gmin = g;
    end
end

sa = sw(imin,1); sb = sw(imin, 2); sc = sw(imin, 3);
Va = Vdc*(2*sa-sb-sc)/3;
Vb = Vdc*(2*sb-sc-sa)/3;
Vc = Vdc*(2*sc-sa-sb)/3;
Vabc = [Va; Vb; Vc];
Vdq = trans*Vabc;
ud_next = Vdq(1, 1);
uq_next = Vdq(2, 1);
